simulink model "P7"  (R2020b)
settings: Solver=VariableStepAuto  StartTime=0.0  StopTime=10.0  RelTol=1e-3
settings Model: Creator=ASUS  LastModifiedBy=ASUS

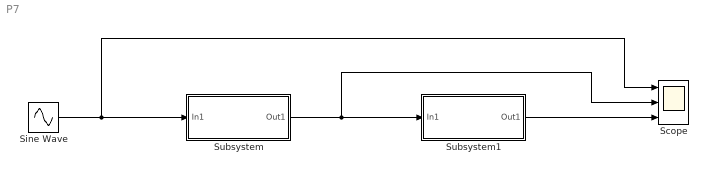
== system P7 ==
  Scope : Scope  NumInputPorts=3
  Sine Wave : Sin  SampleTime=0
  Subsystem : Subsystem
  Subsystem1 : Subsystem
  wires:
  Subsystem1/1(Out1) -> Scope/3
  Sine Wave/1 -> Scope/1, Subsystem/1(In1)
  Subsystem/1(Out1) -> Scope/2, Subsystem1/1(In1)

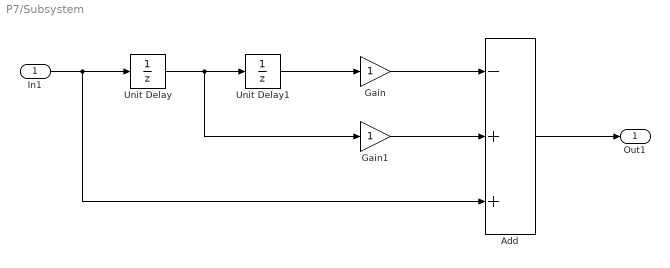
== system P7/Subsystem ==
  In1 : Inport
  Add : Sum  Inputs=-++
  Gain : Gain
  Gain1 : Gain
  Unit Delay : UnitDelay  SampleTime=-1  HasFrameUpgradeWarning=on
  Unit Delay1 : UnitDelay  SampleTime=-1  HasFrameUpgradeWarning=on
  Out1 : Outport
  wires:
  Gain/1 -> Add/1
  Unit Delay1/1 -> Gain/1
  Unit Delay/1 -> Gain1/1, Unit Delay1/1
  In1/1 -> Add/3, Unit Delay/1
  Gain1/1 -> Add/2
  Add/1 -> Out1/1

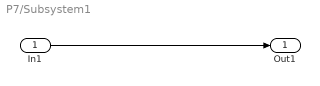
== system P7/Subsystem1 ==
  In1 : Inport
  Out1 : Outport
  wires:
  In1/1 -> Out1/1
